simulink model "Verifica_LQR"  (R2025b)
settings: Solver=VariableStepAuto  StartTime=0.0  StopTime=50.0  RelTol=1e-3
values from neighbouring files (symbols this model uses):
  A = double(subs(A_sym, [x; u], [x_star; u_star]))    [Main_20042026.m]
  B = double(subs(B_sym, [x; u], [x_star; u_star]))    [Main_20042026.m]
  C = double(subs(C_sym, [x; u], [x_star; u_star]))    [Main_20042026.m]
  C_LQR = [0, 1, 0]    [Main_20042026.m]
  D = double(subs(D_sym, [x; u], [x_star; u_star]))    [Main_20042026.m]
  h2_ref_lqr = 2.8    [Main_20042026.m]
  K_LQR_i = K_LQR(:, n+1:end)    [Main_20042026.m]
  K_LQR_x = K_LQR(:, 1:n)    [Main_20042026.m]
settings Model: Creator=salvo  LastModifiedBy=root

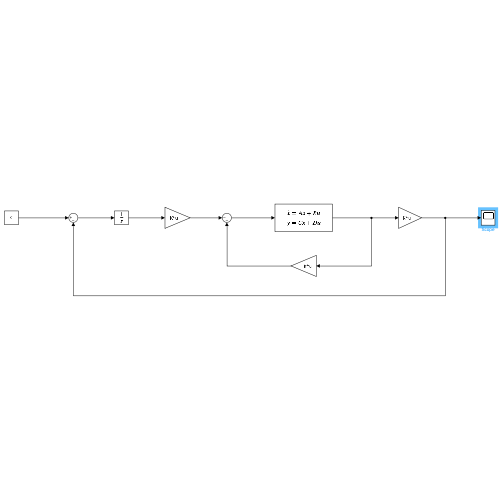
[thumbnail: Simulink's stored preview of the top-level diagram]
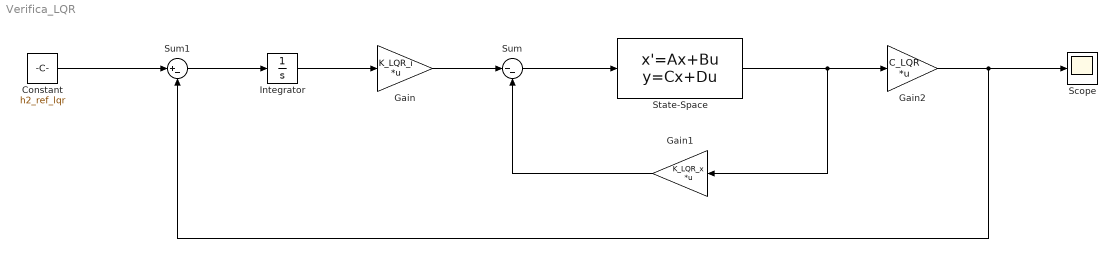
== system Verifica_LQR ==
  Constant : Constant  Value=h2_ref_lqr
  Gain : Gain  Gain=K_LQR_i  Multiplication=Matrix(K*u)
  Gain1 : Gain  Gain=K_LQR_x  Multiplication=Matrix(K*u)
  Gain2 : Gain  Gain=C_LQR  Multiplication=Matrix(K*u)
  Integrator : Integrator
  Scope : Scope
      settings: ActiveDisplayYMinimum=1.8266267665549256  ActiveDisplayYMaximum=3.3536223642774354
  State-Space : StateSpace  A=A  B=B  C=C  D=D  InitialCondition=0
  Sum : Sum  Inputs=|--
  Sum1 : Sum  Inputs=|+-
  wires:
  Sum/1 -> State-Space/1
  State-Space/1 -> Gain1/1, Gain2/1
  Gain2/1 -> Sum1/2, Scope/1
  Gain1/1 -> Sum/2
  Gain/1 -> Sum/1
  Integrator/1 -> Gain/1
  Sum1/1 -> Integrator/1
  Constant/1 -> Sum1/1
